simulink model "plant"  (R2020a)
settings: Solver=VariableStepAuto  StartTime=0.0  StopTime=25.0  RelTol=1e-3
values from neighbouring files (symbols this model uses):
  Ts = 0.1    [main_adaptive_mpc.m]
libraries: mpclib x2, shared6dof x1, sharedtransform x1
settings Model: Creator=Lamarre  LastModifiedBy=Lamarre

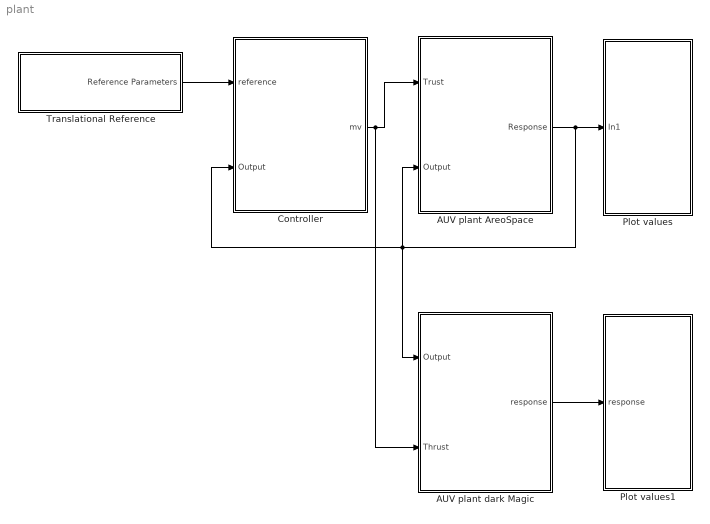
== system plant ==
  AUV plant AreoSpace : Subsystem
  AUV plant dark Magic : Subsystem
  Controller : Subsystem
  Plot values : Subsystem
  Plot values1 : Subsystem
  Translational Reference : Subsystem
  wires:
  Controller/1(mv) -> AUV plant AreoSpace/1(Trust), AUV plant dark Magic/2(Thrust)
  Translational Reference/1(Reference Parameters) -> Controller/1(reference)
  AUV plant AreoSpace/1(Response) -> AUV plant dark Magic/1(Output), Controller/2(Output), AUV plant AreoSpace/2(Output), Plot values/1(In1)
  AUV plant dark Magic/1(response) -> Plot values1/1(response)

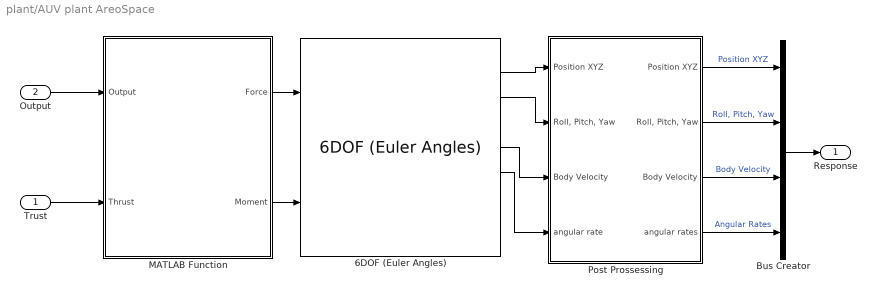
== system plant/AUV plant AreoSpace ==
  Trust : Inport
  Output : Inport  Port=2
  6DOF (Euler Angles) : shared6dof/6DOF (Euler Angles)  units=Metric (MKS)  mtype=Fixed  rep=Euler Angles  xme_0=[0 0 0]  Vm_0=[0 0 0]  eul_0=[0 0 0]  pm_0=[0 0 0]  mass_0=mass  mass_e=0.5  mass_f=2.0  inertia=I  inertia_e=eye(3)  inertia_f=2*eye(3)  k_quat=1.0  vre_flag=on  abi_flag=on  aMode=0  xme_statename=''  Vm_statename=''  eul_statename=''  quat_statename=''  pm_statename=''  mass_statename=''
      settings: SourceProductBaseCode=AE,PW,MT,VE,VP
  Bus Creator : BusCreator  Inputs=4
  MATLAB Function : MATLAB Function  TreatAsAtomicUnit=on
  Post Prossessing : Subsystem
  Response : Outport
  wires:
  MATLAB Function/1(Force) -> 6DOF (Euler Angles)/1
  MATLAB Function/2(Moment) -> 6DOF (Euler Angles)/2
  6DOF (Euler Angles)/2 -> Post Prossessing/1(Position XYZ)
  6DOF (Euler Angles)/3 -> Post Prossessing/2("Roll, Pitch, Yaw")
  Post Prossessing/1("Position XYZ ") -> Bus Creator/1  "Position XYZ"
  6DOF (Euler Angles)/5 -> Post Prossessing/3("Body Velocity ")
  6DOF (Euler Angles)/6 -> Post Prossessing/4(angular rate)
  Post Prossessing/2("Roll, Pitch, Yaw ") -> Bus Creator/2  "Roll, Pitch, Yaw"
  Post Prossessing/3(Body Velocity) -> Bus Creator/3  "Body Velocity"
  Post Prossessing/4(angular rates) -> Bus Creator/4  "Angular Rates"
  Bus Creator/1 -> Response/1
  Output/1 -> MATLAB Function/1(Output)
  Trust/1 -> MATLAB Function/2(Thrust)

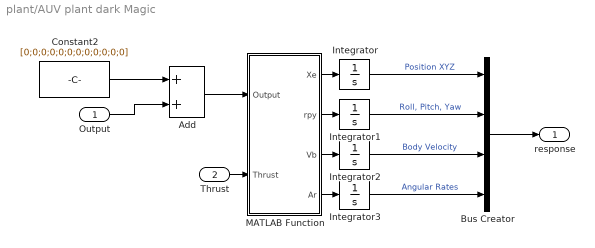
== system plant/AUV plant dark Magic ==
  Output : Inport
  Thrust : Inport  Port=2
  Add : Sum
  Bus Creator : BusCreator  Inputs=4
  Constant2 : Constant  Value=[0;0;0;0;0;0;0;0;0;0;0;0]  VectorParams1D=off
  Integrator{,1..3} (4 alike) : Integrator
  MATLAB Function : MATLAB Function  TreatAsAtomicUnit=on
  response : Outport
  wires:
  Integrator1/1 -> Bus Creator/2  "Roll, Pitch, Yaw"
  Integrator2/1 -> Bus Creator/3  "Body Velocity"
  MATLAB Function/3(Vb) -> Integrator2/1
  MATLAB Function/4(Ar) -> Integrator3/1
  MATLAB Function/2(rpy) -> Integrator1/1
  Bus Creator/1 -> response/1
  Integrator/1 -> Bus Creator/1  "Position XYZ"
  Integrator3/1 -> Bus Creator/4  "Angular Rates"
  MATLAB Function/1(Xe) -> Integrator/1
  Thrust/1 -> MATLAB Function/2(Thrust)
  Constant2/1 -> Add/1
  Output/1 -> Add/2
  Add/1 -> MATLAB Function/1(Output)

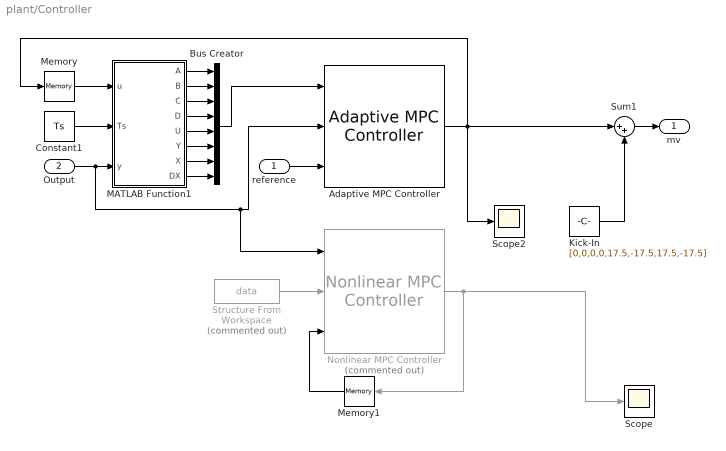
== system plant/Controller ==
  reference : Inport
  Output : Inport  Port=2
  Adaptive MPC Controller : mpclib/Adaptive MPC Controller  SCDEnableBlockLinearizationSpecification=on  mpcobj=mpcobj  enable_value=0  updateMPCinCallerWorkspace=on  md_inport=off  mv_inport=off  uref_inport=off  return_cost=off  return_mvseq=off  return_qpstatus=off  return_xseq=off  return_state=off  return_ovseq=off  state_inport=off  isltv_plant=off  umin_inport=off  umax_inport=off  ymin_inport=off  ymax_inport=off  cc_inport=off  ywt_inport=off  uwt_inport=off  duwt_inport=off  rhoeps_inport=off  pm_inport=off  MaximumP=10  HorizonChoice=FixedHorizon  BlockDataType=double  SampleTimeInherited=off  switch_inport=off
  Bus Creator : BusCreator  Inputs=8
  Constant1 : Constant  Value=Ts
  Kick-In : Constant  Value=[0,0,0,0,17.5,-17.5,17.5,-17.5]
  MATLAB Function1 : MATLAB Function  TreatAsAtomicUnit=on
  Memory : Memory
  Memory1 : Memory
  Nonlinear MPC Controller : mpclib/Nonlinear MPC Controller  Commented=on  SCDEnableBlockLinearizationSpecification=on  nlmpcobj=nlobj  UseObjectTs=on  UseMEX=off  md_enabled=off  mvtarget_enabled=off  param_enabled=off  cost_enabled=off  mvseq_enabled=off  stateseq_enabled=off  ovseq_enabled=off  slack_enabled=off  status_enabled=off  ov_min=off  ov_max=off  mv_min=off  mv_max=off  mvrate_min=off  mvrate_max=off  state_min=off  state_max=off  ov_weight=off  mv_weight=off  mvrate_weight=off  ecr_weight=off  nlp_initialize=off
  Scope : Scope
  Scope2 : Scope
  Structure From Workspace : FromWorkspace  Commented=on  VariableName=data
  Sum1 : Sum  Inputs=|++
  mv : Outport
  wires:
  MATLAB Function1/5(U) -> Bus Creator/5
  Bus Creator/1 -> Adaptive MPC Controller/1
  MATLAB Function1/7(X) -> Bus Creator/7
  MATLAB Function1/2(B) -> Bus Creator/2
  Adaptive MPC Controller/1 -> Scope2/1, Sum1/1, Memory/1
  MATLAB Function1/3(C) -> Bus Creator/3
  MATLAB Function1/1(A) -> Bus Creator/1
  MATLAB Function1/4(D) -> Bus Creator/4
  MATLAB Function1/8(DX) -> Bus Creator/8
  MATLAB Function1/6(Y) -> Bus Creator/6
  Constant1/1 -> MATLAB Function1/2(Ts)
  Kick-In/1 -> Sum1/2
  Memory/1 -> MATLAB Function1/1(u)
  Output/1 -> Nonlinear MPC Controller/1, Adaptive MPC Controller/2, MATLAB Function1/3(y)
  Nonlinear MPC Controller/1 -> Memory1/1, Scope/1
  Memory1/1 -> Nonlinear MPC Controller/3
  Sum1/1 -> mv/1
  reference/1 -> Adaptive MPC Controller/3
  Structure From Workspace/1 -> Nonlinear MPC Controller/2

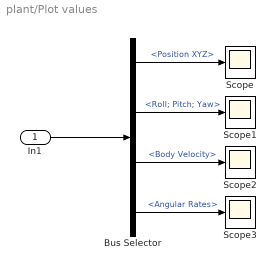
== system plant/Plot values ==
  In1 : Inport
  Bus Selector : BusSelector  OutputSignals=Position XYZ,Roll; Pitch; Yaw,Body Velocity,Angular Rates
  Scope{,1..3} (4 alike) : Scope
  wires:
  Bus Selector/4 -> Scope3/1  "<Angular Rates>"
  In1/1 -> Bus Selector/1
  Bus Selector/1 -> Scope/1  "<Position XYZ>"
  Bus Selector/2 -> Scope1/1  "<Roll; Pitch; Yaw>"
  Bus Selector/3 -> Scope2/1  "<Body Velocity>"

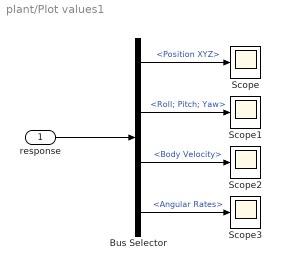
== system plant/Plot values1 ==
  response : Inport
  Bus Selector : BusSelector  OutputSignals=Position XYZ,Roll; Pitch; Yaw,Body Velocity,Angular Rates
  Scope{,1..3} (4 alike) : Scope
  wires:
  Bus Selector/4 -> Scope3/1  "<Angular Rates>"
  response/1 -> Bus Selector/1
  Bus Selector/1 -> Scope/1  "<Position XYZ>"
  Bus Selector/2 -> Scope1/1  "<Roll; Pitch; Yaw>"
  Bus Selector/3 -> Scope2/1  "<Body Velocity>"

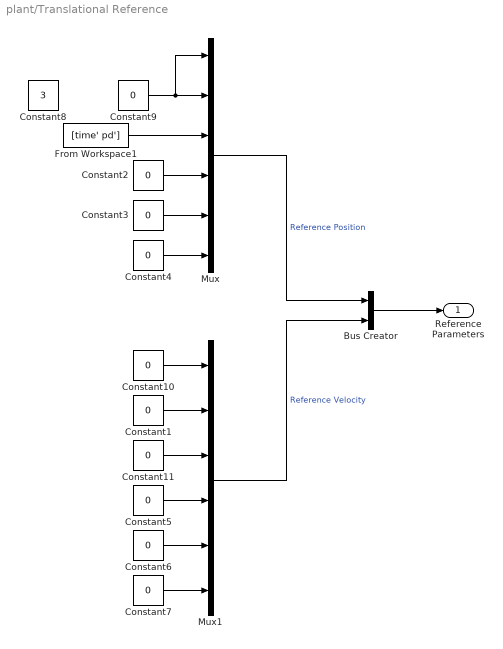
== system plant/Translational Reference ==
  Bus Creator : BusCreator  Inputs=2
  Constant{1..7,9..11} (10 alike) : Constant  Value=0
  Constant8 : Constant  Value=3
  From Workspace1 : FromWorkspace  VariableName=[time' pd']
  Mux : Mux  Inputs=6
  Mux1 : Mux  Inputs=6
  Reference Parameters : Outport  VectorParamsAs1DForOutWhenUnconnected=off
  wires:
  Mux/1 -> Bus Creator/1  "Reference Position"
  Mux1/1 -> Bus Creator/2  "Reference Velocity"
  Bus Creator/1 -> Reference Parameters/1
  Constant1/1 -> Mux1/2
  Constant2/1 -> Mux/4
  Constant3/1 -> Mux/5
  Constant4/1 -> Mux/6
  Constant6/1 -> Mux1/5
  Constant7/1 -> Mux1/6
  Constant5/1 -> Mux1/4
  Constant10/1 -> Mux1/1
  Constant11/1 -> Mux1/3
  Constant9/1 -> Mux/1, Mux/2
  From Workspace1/1 -> Mux/3

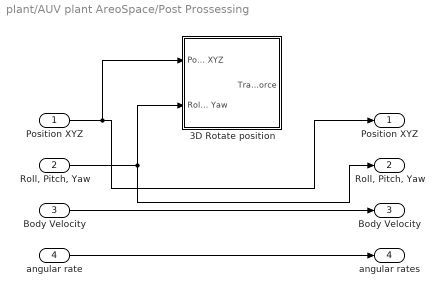
== system plant/AUV plant AreoSpace/Post Prossessing ==
  Position XYZ : Inport
  "Roll, Pitch, Yaw" : Inport  Port=2
  "Body Velocity " : Inport  Port=3
  angular rate : Inport  Port=4
  3D Rotate position : Subsystem
  "Position XYZ " : Outport
  "Roll, Pitch, Yaw " : Outport  Port=2
  Body Velocity : Outport  Port=3
  angular rates : Outport  Port=4
  wires:
  "Roll, Pitch, Yaw"/1 -> "Roll, Pitch, Yaw "/1, 3D Rotate position/2("Roll, Pitch, Yaw")
  "Body Velocity "/1 -> Body Velocity/1
  angular rate/1 -> angular rates/1
  Position XYZ/1 -> 3D Rotate position/1(Position XYZ), "Position XYZ "/1

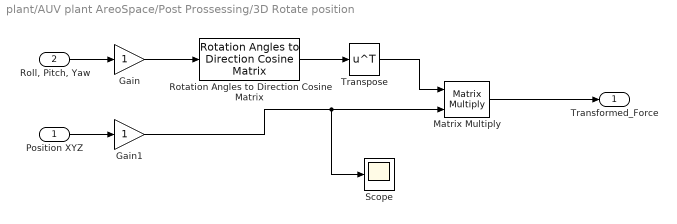
== system plant/AUV plant AreoSpace/Post Prossessing/3D Rotate position ==
  Position XYZ : Inport
  "Roll, Pitch, Yaw" : Inport  Port=2
  Gain : Gain
  Gain1 : Gain
  Matrix Multiply : Product  Multiplication=Matrix(*)
  Rotation Angles to Direction Cosine Matrix : sharedtransform/Rotation Angles to Direction Cosine Matrix  rotationOrder=XYZ  aMode=aMode
      settings: SourceProductBaseCode=AE,PW,MT,VE,VP
  Scope : Scope
  Transpose : Math  Operator=transpose  SignedPower=on  SaturateOnIntegerOverflow=on
  "Transformed_Force " : Outport  VectorParamsAs1DForOutWhenUnconnected=off
  wires:
  Matrix Multiply/1 -> "Transformed_Force "/1
  Rotation Angles to Direction Cosine Matrix/1 -> Transpose/1
  Transpose/1 -> Matrix Multiply/1
  Gain/1 -> Rotation Angles to Direction Cosine Matrix/1
  Gain1/1 -> Scope/1, Matrix Multiply/2
  Position XYZ/1 -> Gain1/1
  "Roll, Pitch, Yaw"/1 -> Gain/1

== matlab function plant/AUV plant AreoSpace/MATLAB Function ==
  data: Output input; Force output; Thrust input; Moment output
function [Force,Moment] = Calculate_Forces_and_Torques(Output,Thrust)
Dynamics=AUVForceMoments(Output,Thrust);
Force=Dynamics(1:3);
Moment= Dynamics(4:6);

== matlab function plant/AUV plant dark Magic/MATLAB Function ==
  data: Output input; Thrust input; Xe output; rpy output; Vb output; Ar output
function [Xe,rpy,Vb,Ar ] = fcn(Output,Thrust)

xdot = AUVStateSimFcn(Output,Thrust);
Xe = xdot(1:3);
rpy = xdot(4:6);
Vb = xdot(7:9);
Ar = xdot(10:12);

== matlab function plant/Controller/MATLAB Function1 ==
  data: u input; Ts input; y input; A output; B output; C output; D output; U output; Y output; X output; DX output
function [A,B,C,D,U,Y,X,DX] = Plant(u,Ts,y)
% Lineariser le model dynamique

%x=[y(4:5,1);y(7:12,1)];
%x(5)=x(5)-.85;
[Ac, Bc, Cc, Dc]=AUVStateJacobianFcn(y,u);
% Generate discrete-time model

%  nx = size(Ac,1);
%  nu = size(Bc,2);
%cplant=ss(Ac,Bc,Cc,Dc);
%plant=c2d(cplant,Ts,'zoh');

nx = size(Ac,1);
nu = size(Bc,2);
M = expm([[Ac Bc]*Ts; zeros(nu,nu+nx)]);
A = M(1:nx,1:nx);
B = M(1:nx,nx+1:nx+nu);
C = Cc;
D = Dc;
 %xx=[X(4:5,1);X(7:12)];

% cplant=ss(Ac,Bc,Cc,Dc);
% plant=c2d(cplant,Ts,'zoh');
%plant=ss(A,B,C,D,Ts);

% Nominal conditions for discrete-time plant
U=u.';
Y=(Cc*y + Dc*u).';
X=y.';
DX=(A*y+B*u-y).';
